simulink model "untitled_2_2"  (R2025b)
settings: Solver=ode45  StartTime=0.0  StopTime=5  RelTol=1e-3  EnableMultiTasking=on
settings Model: Creator=115326  LastModifiedBy=Lenovo
settings SolverCC: AlgebraicLoopSolver=TrustRegion
settings DataIOCC: LimitDataPoints=on  SaveFormat=Array  SignalLoggingSaveFormat=ModelDataLogs  ReturnWorkspaceOutputs=off
settings OptimizationCC: ExpressionDepthLimit=2147483647.0  LifeSpan=inf
settings DebuggingCC: UnderspecifiedInitializationDetection=Classic  MergeDetectMultiDrivingBlocksExec=none  SolverPrmCheckMsg=warning  FcnCallInpInsideContextMsg=warning  UnconnectedInputMsg=warning  UnconnectedOutputMsg=warning  UnconnectedLineMsg=warning  StateNameClashWarn=warning  SFUnexpectedBacktrackingDiag=warning  SFNoUnconditionalDefaultTransitionDiag=warning  SFExecutionAtInitializationDiag=none  ArithmeticOperatorsInVariantConditions=warning
settings HardwareCC: ProdBitPerPointer=32.0  ProdBitPerSizeT=32.0  ProdBitPerPtrDiffT=32.0  ProdLargestAtomicFloat=None  ProdIntDivRoundTo=Undefined  ProdEndianess=Unspecified  ProdWordSize=32.0  ProdHWDeviceType=32-bit Generic
settings ModelReferenceCC: PropagateSignalLabelsOutOfModel=off
settings SFSimCC: SimUseLocalCustomCode=off  CustomCodeUndefinedFunction=UseInterfaceOnly
settings RTWCC: RTWUseLocalCustomCode=off  GPUComputeCapability=3.5
settings CodeAppCC: StateflowObjectComments=on
settings GRTTargetCC: TargetLangStandard=C89/C90 (ANSI)  CombineOutputUpdateFcns=off  GRTInterface=on
settings ConfigComp: CovMetricSettings=dw  CovSaveCumulativeToWorkspaceVar=on  CovSaveSingleToWorkspaceVar=on  CovExternalEMLEnable=off

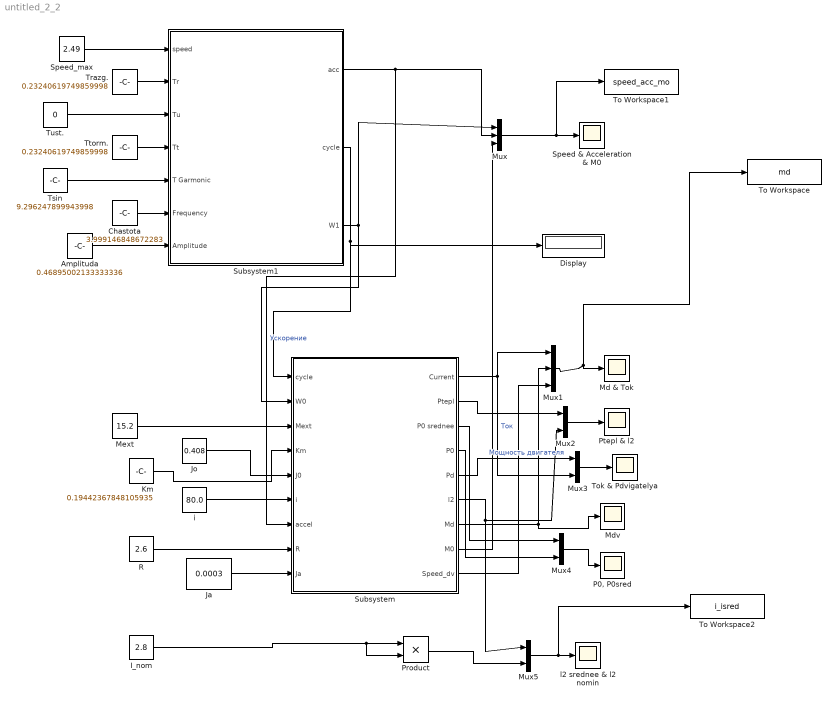
== system untitled_2_2 ==
  Amplituda : Constant  Value=0.46895002133333336
  Chastota : Constant  Value=3.999146848672283
  Display : Display
  I_nom : Constant  Value=2.8
  Ja : Constant  Value=0.0003
  Jo : Constant  Value=0.408
  Km : Constant  Value=0.19442367848105935
  Md & Tok : Scope
      settings: ActiveDisplayYMinimum=-1566.8844359938671  ActiveDisplayYMaximum=3677.2829840417808  DataLoggingVariableName=ScopeData2
  Mdv : Scope
      settings: ActiveDisplayYMinimum=-1  ActiveDisplayYMaximum=1  DataLoggingVariableName=ScopeData5
  Mext : Constant  Value=15.2
  Mux : Mux  Inputs=3
  Mux1 : Mux  Inputs=3
  Mux{2..5} (4 alike) : Mux  Inputs=2
  "P0, P0sred" : Scope
      settings: ActiveDisplayYMinimum=-1  ActiveDisplayYMaximum=1  DataLoggingVariableName=ScopeData4
  Product : Product  RndMeth=Zero
  Ptepl & l2 : Scope
      settings: ActiveDisplayYMinimum=-1  ActiveDisplayYMaximum=1  DataLoggingVariableName=ScopeData3
  R : Constant  Value=2.6
  Speed & Acceleration & M0 : Scope
      settings: ActiveDisplayYMinimum=-22.716029124999991  ActiveDisplayYMaximum=133.25426212499997
  Speed_max : Constant  Value=2.49
  Subsystem : Subsystem
  Subsystem1 : Subsystem
  To Workspace : ToWorkspace  VariableName=md  SaveFormat=Structure With Time  SampleTime=-1
  To Workspace1 : ToWorkspace  VariableName=speed_acc_mo  SaveFormat=Structure With Time  SampleTime=-1
  To Workspace2 : ToWorkspace  VariableName=i_isred  SaveFormat=Structure With Time  SampleTime=-1
  Tok & Pdvigatelya : Scope
      settings: ActiveDisplayYMinimum=-302.32374128571354  ActiveDisplayYMaximum=724.92654128570734
  Trazg. : Constant  Value=0.23240619749859998
  Tsin : Constant  Value=9.296247899943998
  Ttorm. : Constant  Value=0.23240619749859998
  Tust. : Constant  Value=0
  i : Constant  Value=80.0
  l2 srednee & l2 nomin : Scope
      settings: ActiveDisplayYMinimum=-17.99981228734644  ActiveDisplayYMaximum=161.9999791430385  DataLoggingVariableName=ScopeData6
  wires:
  Trazg./1 -> Subsystem1/2(Tr)
  Tust./1 -> Subsystem1/3(Tu)
  Ttorm./1 -> Subsystem1/4(Tt)
  Tsin/1 -> Subsystem1/5(T Garmonic)
  Chastota/1 -> Subsystem1/6(Frequency)
  Amplituda/1 -> Subsystem1/7(Amplitude)
  Subsystem1/3(W1) -> Subsystem/2(W0), Mux/1
  Subsystem1/1(acc) -> Mux/2, Subsystem/7(accel)  "Ускорение"
  Subsystem1/2(cycle) -> Subsystem/1(cycle), Display/1
  Mext/1 -> Subsystem/3(Mext)
  R/1 -> Subsystem/8(R)
  Jo/1 -> Subsystem/5(J0)
  i/1 -> Subsystem/6(i)
  Ja/1 -> Subsystem/9(Ja)
  Subsystem/8(M0) -> Mux/3
  Subsystem/1(Current) -> Mux1/1, Mux3/2  "Ток"
  Subsystem/7(Md) -> Mdv/1, Mux1/2
  Subsystem/5(Pd) -> Mux3/1  "Мощность двигателя"
  Subsystem/2(Ptepl) -> Mux2/1
  Subsystem/6(l2) -> Mux2/2, Mux5/1
  Subsystem/4(P0) -> Mux4/2
  Subsystem/3(P0 srednee) -> Mux4/1
  Mux4/1 -> "P0, P0sred"/1
  Mux3/1 -> Tok & Pdvigatelya/1
  Mux1/1 -> To Workspace/1, Md & Tok/1
  Mux/1 -> To Workspace1/1, Speed & Acceleration & M0/1
  Mux2/1 -> Ptepl & l2/1
  I_nom/1 -> Product/1, Product/2
  Product/1 -> Mux5/2
  Mux5/1 -> To Workspace2/1, l2 srednee & l2 nomin/1
  Km/1 -> Subsystem/4(Km)
  Speed_max/1 -> Subsystem1/1(speed)
  Subsystem/9(Speed_dv) -> Mux1/3

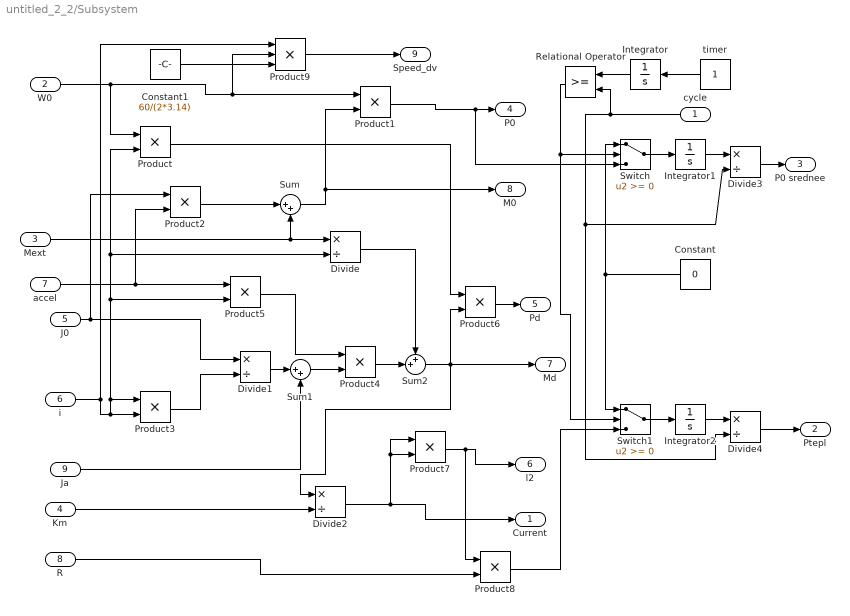
== system untitled_2_2/Subsystem ==
  cycle : Inport
  W0 : Inport  Port=2
  Mext : Inport  Port=3
  Km : Inport  Port=4
  J0 : Inport  Port=5
  i : Inport  Port=6
  accel : Inport  Port=7
  R : Inport  Port=8
  Ja : Inport  Port=9
  Constant : Constant  Value=0
  Constant1 : Constant  Value=60/(2*3.14)
  Divide{,1..4} (5 alike) : Product  Inputs=*/
  Integrator : Integrator
  Integrator1 : Integrator
  Integrator2 : Integrator
  Product{,1..8} (9 alike) : Product  RndMeth=Zero
  Product9 : Product  Inputs=3  RndMeth=Zero
  Relational Operator : RelationalOperator  OutDataTypeStr=boolean  InputSameDT=off
  Sum : Sum  Inputs=|++
  Sum1 : Sum  Inputs=|++
  Sum2 : Sum  Inputs=++|
  Switch : Switch  SaturateOnIntegerOverflow=off  InputSameDT=off
  Switch1 : Switch  SaturateOnIntegerOverflow=off  InputSameDT=off
  timer : Constant
  Current : Outport
  Ptepl : Outport  Port=2
  P0 srednee : Outport  Port=3
  P0 : Outport  Port=4
  Pd : Outport  Port=5
  l2 : Outport  Port=6
  Md : Outport  Port=7
  M0 : Outport  Port=8
  Speed_dv : Outport  Port=9
  wires:
  W0/1 -> Product9/2, Product1/1, Product/1
  Product2/1 -> Sum/1
  i/1 -> Product9/1, Product3/2, Product3/1, Product5/2, Product/2, Divide/2
  J0/1 -> Divide1/1, Product2/1
  Product3/1 -> Divide1/2
  Divide1/1 -> Sum1/1
  Ja/1 -> Sum1/2
  Sum1/1 -> Product4/2
  Product4/1 -> Sum2/2
  Mext/1 -> Divide/1, Sum/2
  accel/1 -> Product5/1, Product2/2
  Sum/1 -> Product1/2, M0/1
  Product/1 -> Product6/1
  Km/1 -> Divide2/2
  Divide2/1 -> Current/1, Product7/2, Product7/1
  Product7/1 -> l2/1, Product8/1
  R/1 -> Product8/2
  Sum2/1 -> Md/1, Product6/2, Divide2/1
  Product6/1 -> Pd/1
  Product1/1 -> P0/1, Switch/3
  Integrator/1 -> Relational Operator/1
  Relational Operator/1 -> Switch1/2, Switch/2
  Product8/1 -> Switch1/3
  Switch1/1 -> Integrator2/1
  Integrator2/1 -> Divide4/1
  cycle/1 -> Relational Operator/2, Divide4/2, Divide3/2
  Integrator1/1 -> Divide3/1
  Constant/1 -> Switch/1, Switch1/1
  Switch/1 -> Integrator1/1
  timer/1 -> Integrator/1
  Divide4/1 -> Ptepl/1
  Divide3/1 -> P0 srednee/1
  Divide/1 -> Sum2/1
  Product5/1 -> Product4/1
  Constant1/1 -> Product9/3
  Product9/1 -> Speed_dv/1

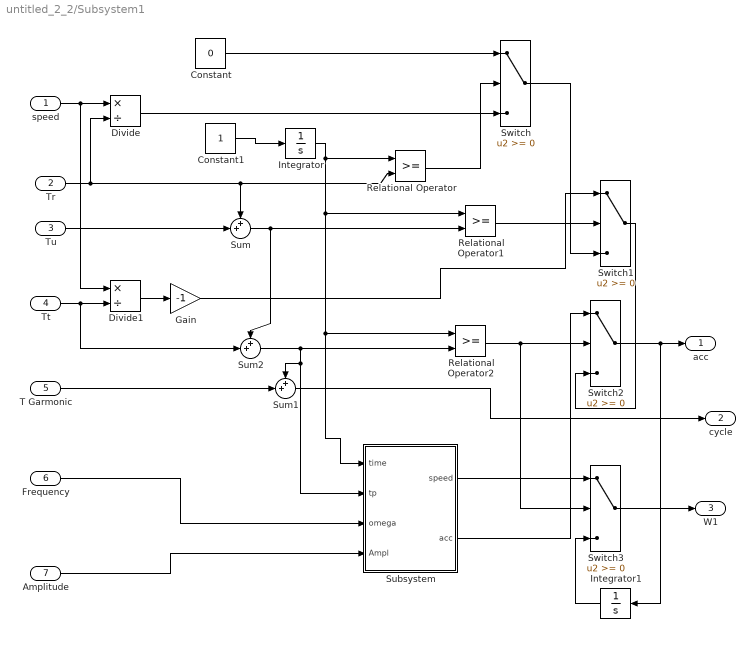
== system untitled_2_2/Subsystem1 ==
  speed : Inport
  Tr : Inport  Port=2
  Tu : Inport  Port=3
  Tt : Inport  Port=4
  T Garmonic : Inport  Port=5
  Frequency : Inport  Port=6
  Amplitude : Inport  Port=7
  Constant : Constant  Value=0
  Constant1 : Constant
  Divide : Product  Inputs=*/
  Divide1 : Product  Inputs=*/
  Gain : Gain  Gain=-1
  Integrator : Integrator
  Integrator1 : Integrator
  Relational Operator : RelationalOperator  OutDataTypeStr=boolean  InputSameDT=off
  Relational Operator1 : RelationalOperator  OutDataTypeStr=boolean  InputSameDT=off
  Relational Operator2 : RelationalOperator  OutDataTypeStr=boolean  InputSameDT=off
  Subsystem : Subsystem
  Sum : Sum  Inputs=++|
  Sum1 : Sum  Inputs=++|
  Sum2 : Sum  Inputs=++|
  Switch{,1..3} (4 alike) : Switch  SaturateOnIntegerOverflow=off  InputSameDT=off
  acc : Outport
  cycle : Outport  Port=2
  W1 : Outport  Port=3
  wires:
  speed/1 -> Divide/1, Divide1/1
  Constant/1 -> Switch/1
  Divide/1 -> Switch/3
  Tt/1 -> Divide1/2, Sum2/2
  Tr/1 -> Relational Operator/2, Sum/1, Divide/2
  Tu/1 -> Sum/2
  Sum/1 -> Relational Operator1/2, Sum2/1
  Relational Operator/1 -> Switch/2
  Relational Operator1/1 -> Switch1/2
  Divide1/1 -> Gain/1
  Gain/1 -> Switch1/1
  Sum2/1 -> Relational Operator2/2, Subsystem/2(tp), Sum1/1
  Relational Operator2/1 -> Switch2/2, Switch3/2
  Switch1/1 -> Switch2/3
  Switch/1 -> Switch1/3
  T Garmonic/1 -> Sum1/2
  Sum1/1 -> cycle/1
  Switch2/1 -> acc/1, Integrator1/1
  Constant1/1 -> Integrator/1
  Frequency/1 -> Subsystem/3(omega)
  Amplitude/1 -> Subsystem/4(Ampl)
  Integrator/1 -> Subsystem/1(time), Relational Operator2/1, Relational Operator1/1, Relational Operator/1
  Subsystem/1(speed) -> Switch3/1
  Subsystem/2(acc) -> Switch2/1
  Integrator1/1 -> Switch3/3
  Switch3/1 -> W1/1

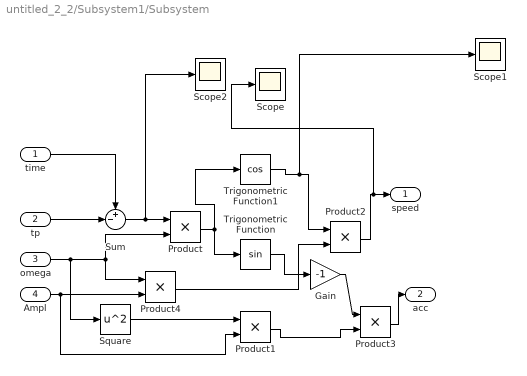
== system untitled_2_2/Subsystem1/Subsystem ==
  time : Inport
  tp : Inport  Port=2
  omega : Inport  Port=3
  Ampl : Inport  Port=4
  Gain : Gain  Gain=-1
  Product{,1..3} (4 alike) : Product  RndMeth=Zero
  Product4 : Product
  Scope : Scope
      settings: ActiveDisplayYMinimum=-0.090563234504098727  ActiveDisplayYMaximum=0.41573544394957596  DataLoggingVariableName=ScopeData7
  Scope1 : Scope
      settings: ActiveDisplayYMinimum=-1  ActiveDisplayYMaximum=1  DataLoggingVariableName=ScopeData8
  Scope2 : Scope
      settings: ActiveDisplayYMinimum=-1  ActiveDisplayYMaximum=1  DataLoggingVariableName=ScopeData9
  Square : Math  Operator=square
  Sum : Sum  Inputs=+-|
  Trigonometric Function : Trigonometry
  Trigonometric Function1 : Trigonometry  Operator=cos
  speed : Outport
  acc : Outport  Port=2
  wires:
  tp/1 -> Sum/2
  time/1 -> Sum/1
  Sum/1 -> Scope2/1, Product/1
  omega/1 -> Product/2, Product4/1, Square/1
  Ampl/1 -> Product1/2, Product4/2
  Product/1 -> Trigonometric Function1/1, Trigonometric Function/1
  Product2/1 -> Scope/1, speed/1
  Product3/1 -> acc/1
  Product4/1 -> Product2/2
  Square/1 -> Product1/1
  Trigonometric Function1/1 -> Scope1/1, Product2/1
  Product1/1 -> Product3/2
  Trigonometric Function/1 -> Gain/1
  Gain/1 -> Product3/1
